simulink model "temperatura_testes_anti_windup"  (R2020a)
settings: Solver=VariableStepAuto  StartTime=0.0  StopTime=100000  RelTol=1e-3
settings Model: Creator=gabriel  LastModifiedBy=gabriel

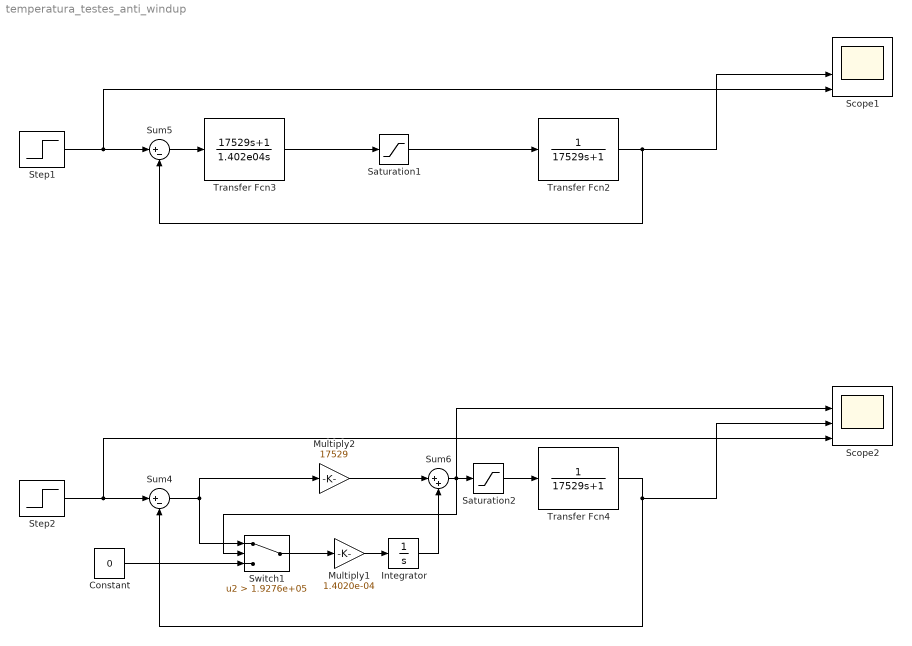
== system temperatura_testes_anti_windup ==
  Constant : Constant  Value=0
  Integrator : Integrator
  Multiply1 : Gain  Gain=1.4020e-04
  Multiply2 : Gain  Gain=17529
  Saturation1 : Saturate  UpperLimit=4  LowerLimit=-0.6
  Saturation2 : Saturate  UpperLimit=4  LowerLimit=-0.6
  Scope1 : Scope  NumInputPorts=4
  Scope2 : Scope  NumInputPorts=4
  Step1 : Step  Time=100  SampleTime=0
  Step2 : Step  Time=100  SampleTime=0
  Sum4 : Sum  Inputs=|+-
  Sum5 : Sum  Inputs=|+-
  Sum6 : Sum  Inputs=|++
  Switch1 : Switch  Criteria=u2 > Threshold  Threshold=1.9276e+05
  Transfer Fcn2 : TransferFcn  Denominator=[17529 1]
  Transfer Fcn3 : TransferFcn  Numerator=[17529 1]  Denominator=[1.402e04 0]
  Transfer Fcn4 : TransferFcn  Denominator=[17529 1]
  wires:
  Saturation1/1 -> Transfer Fcn2/1
  Transfer Fcn2/1 -> Scope1/3, Sum5/2
  Step1/1 -> Scope1/4, Sum5/1
  Sum5/1 -> Transfer Fcn3/1
  Transfer Fcn3/1 -> Saturation1/1
  Step2/1 -> Scope2/4, Sum4/1
  Transfer Fcn4/1 -> Scope2/3, Sum4/2
  Sum4/1 -> Multiply2/1, Switch1/1
  Saturation2/1 -> Transfer Fcn4/1
  Multiply1/1 -> Integrator/1
  Sum6/1 -> Switch1/2, Saturation2/1, Scope2/2
  Integrator/1 -> Sum6/2
  Switch1/1 -> Multiply1/1
  Multiply2/1 -> Sum6/1
  Constant/1 -> Switch1/3
